simulink library "Lib_Turbo_Duct_TMATS_org"  (Simulink 10.0)
settings: Solver=ode45  StartTime=0.0  StopTime=10.0  RelTol=1e-3  EnableMultiTasking=on
Description:
  | Thomas Modules
settings Model: Creator=jwchapm2  LastModifiedBy=bhisma

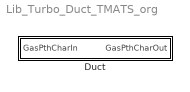
== system Lib_Turbo_Duct_TMATS_org ==
  Duct : Subsystem  mask(T-MATS: Duct Library Block){dP_M=0.005}
      mask prompts: dP_M "dP_M - Delta Pressure [frac lost]"
      mask help: This block simulates the performance of a duct using basic fluid dynamic equations and properties.
      mask Help: web(which('Turbo_TMATS_Dct.html'),'-helpbrowser')

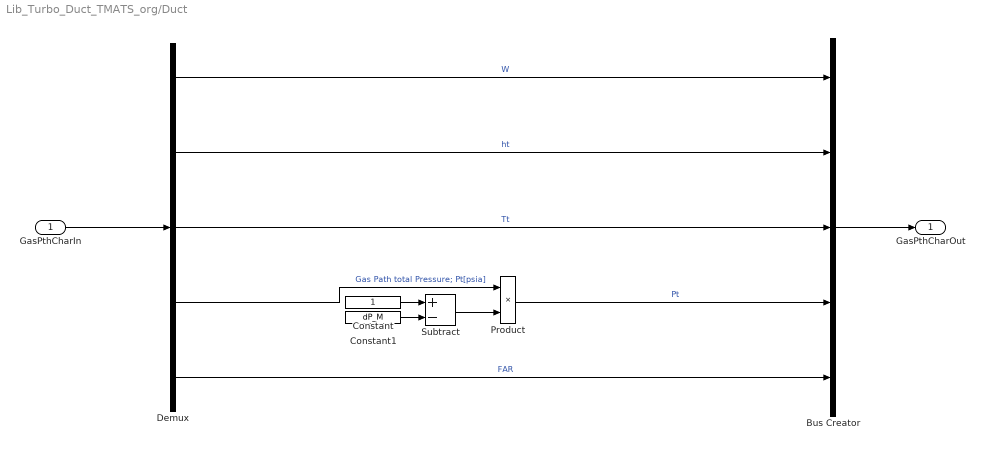
== system Lib_Turbo_Duct_TMATS_org/Duct ==
  GasPthCharIn : Inport
  Bus Creator : BusCreator  Inputs=5
  Constant : Constant
  Constant1 : Constant  Value=dP_M
  Demux : Demux  Outputs=5
  Product : Product  RndMeth=Zero
  Subtract : Sum  Inputs=+-
  GasPthCharOut : Outport
  wires:
  Constant/1 -> Subtract/1
  Constant1/1 -> Subtract/2
  Demux/1 -> Bus Creator/1  "W"
  Demux/5 -> Bus Creator/5  "FAR"
  Demux/3 -> Bus Creator/3  "Tt"
  GasPthCharIn/1 -> Demux/1
  Bus Creator/1 -> GasPthCharOut/1
  Product/1 -> Bus Creator/4  "Pt"
  Demux/4 -> Product/1  "Gas Path total Pressure; Pt[psia]"
  Subtract/1 -> Product/2
  Demux/2 -> Bus Creator/2  "ht"
